simulink model "controlPosicion_2018a"  (R2018a)
settings: Solver=VariableStepAuto  StartTime=0.0  StopTime=18  RelTol=1e-3
values from neighbouring files (symbols this model uses):
  kp = 3    [Calculo_Tau_RR.m]
  kv = 2*sqrt(kp)    [Calculo_Tau_RR.m]
libraries: roblocks x5, simulink x1
settings Model: Creator=Marcelo  LastModifiedBy=rochi
settings DataIOCC: ReturnWorkspaceOutputs=on
settings SFSimCC: SimUseLocalCustomCode=on
settings RTWCC: RTWUseLocalCustomCode=on

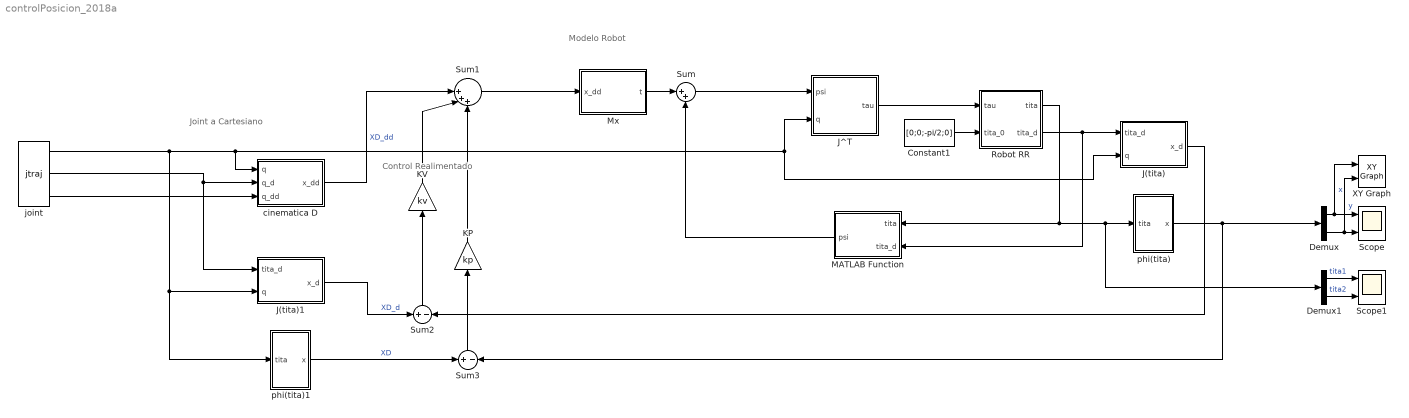
== system controlPosicion_2018a ==
  note: Control Realimentado
  note: Joint a Cartesiano
  note: Modelo Robot
  Constant1 : Constant  Value=[0;0;-pi/2;0]
  Demux : Demux  Outputs=2
  Demux1 : Demux  Outputs=2
  J(tita) : MATLAB Function  TreatAsAtomicUnit=on
  J(tita)1 : MATLAB Function  TreatAsAtomicUnit=on
  J^T : MATLAB Function  TreatAsAtomicUnit=on
  KP : Gain  Gain=kp
  KV : Gain  Gain=kv
  MATLAB Function : MATLAB Function  TreatAsAtomicUnit=on
  Mx : MATLAB Function  TreatAsAtomicUnit=on
  Robot RR : Subsystem
  Scope : Scope  NumInputPorts=2
  Scope1 : Scope  NumInputPorts=2
  Sum : Sum  Inputs=|++
  Sum1 : Sum  Inputs=||+++
  Sum2 : Sum  Inputs=+|-
  Sum3 : Sum  Inputs=+|-
  XY Graph : simulink/Sinks/XY Graph  xmin=-2  xmax=2  ymin=-2  ymax=2  st=-1
  cinematica D : MATLAB Function  TreatAsAtomicUnit=on
  joint : roblocks/Toolbox/jtraj  q0=[0 -pi/2]  qf=[pi/2 -pi/2]  tmax=10  ts=0.02
  phi(tita) : Subsystem
  phi(tita)1 : Subsystem
  wires:
  Robot RR/2(tita_d) -> J(tita)/1(tita_d), MATLAB Function/2(tita_d)
  MATLAB Function/1(psi) -> Sum/2
  KP/1 -> Sum1/3
  KV/1 -> Sum1/2
  Sum3/1 -> KP/1
  Sum2/1 -> KV/1
  phi(tita)/1(x) -> Sum3/2, Demux/1
  Demux/1 -> XY Graph/1, Scope/1  "x"
  Demux/2 -> XY Graph/2, Scope/2  "y"
  Constant1/1 -> Robot RR/2(tita_0)
  Mx/1(t) -> Sum/1
  Sum1/1 -> Mx/1(x_dd)
  Demux1/2 -> Scope1/2  "tita2"
  Demux1/1 -> Scope1/1  "tita1"
  J^T/1(tau) -> Robot RR/1(tau)
  Sum/1 -> J^T/1(psi)
  J(tita)/1(x_d) -> Sum2/2
  Robot RR/1(tita) -> Demux1/1, phi(tita)/1(tita), MATLAB Function/1(tita)
  joint/1 -> cinematica D/1(q), J(tita)/2(q), J^T/2(q), phi(tita)1/1(tita), J(tita)1/2(q)
  phi(tita)1/1(x) -> Sum3/1  "XD"
  J(tita)1/1(x_d) -> Sum2/1  "XD_d"
  joint/2 -> cinematica D/2(q_d), J(tita)1/1(tita_d)
  cinematica D/1(x_dd) -> Sum1/1  "XD_dd"
  joint/3 -> cinematica D/3(q_dd)

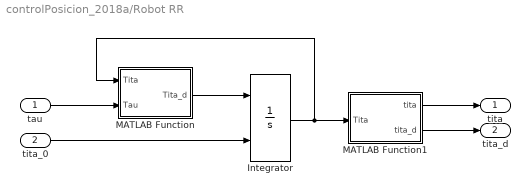
== system controlPosicion_2018a/Robot RR ==
  tau : Inport
  tita_0 : Inport  Port=2
  Integrator : Integrator  InitialConditionSource=external
  MATLAB Function : MATLAB Function  TreatAsAtomicUnit=on
  MATLAB Function1 : MATLAB Function  TreatAsAtomicUnit=on
  tita : Outport
  tita_d : Outport  Port=2
  wires:
  tau/1 -> MATLAB Function/2(Tau)
  MATLAB Function/1(Tita_d) -> Integrator/1
  tita_0/1 -> Integrator/2
  Integrator/1 -> MATLAB Function1/1(Tita), MATLAB Function/1(Tita)
  MATLAB Function1/1(tita) -> tita/1
  MATLAB Function1/2(tita_d) -> tita_d/1

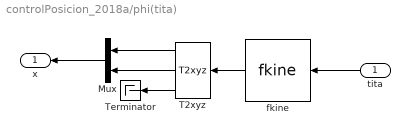
== system controlPosicion_2018a/phi(tita) ==
  tita : Inport
  Mux : Mux  Inputs=2
  T2xyz : roblocks/Toolbox/T2xyz
  Terminator : Terminator
  fkine : roblocks/Arm/fkine  robot=Robot
  x : Outport
  wires:
  T2xyz/2 -> Mux/2
  Mux/1 -> x/1
  fkine/1 -> T2xyz/1
  tita/1 -> fkine/1
  T2xyz/1 -> Mux/1
  T2xyz/3 -> Terminator/1

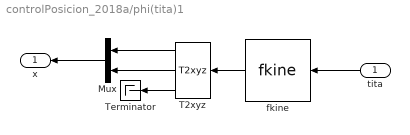
== system controlPosicion_2018a/phi(tita)1 ==
  tita : Inport
  Mux : Mux  Inputs=2
  T2xyz : roblocks/Toolbox/T2xyz
  Terminator : Terminator
  fkine : roblocks/Arm/fkine  robot=Robot
  x : Outport
  wires:
  T2xyz/2 -> Mux/2
  Mux/1 -> x/1
  fkine/1 -> T2xyz/1
  tita/1 -> fkine/1
  T2xyz/1 -> Mux/1
  T2xyz/3 -> Terminator/1

== matlab function controlPosicion_2018a/MATLAB Function ==
  data: tita input; psi output; tita_d input
function psi = f(tita,tita_d)

psi1 = tita_d(1);
psi2 = tita_d(2);

psi = [psi1;psi2];

== matlab function controlPosicion_2018a/J^T ==
  data: psi input; tau output; q input
function tau = fcn(psi,q)

th2 = q(2);
J = [sin(th2) 0; cos(th2)+1 1];

tau = (J')*psi;

== matlab function controlPosicion_2018a/Robot RR/MATLAB Function ==
  data: Tita input; Tita_d output; Tau input
function Tita_d = fcn(Tita,Tau)

titad1 = Tita(2);
titadd1 = Tau(1)-Tita(2);
titad2 = Tau(2);
titadd2 = 0;

Tita_d = [titad1;titadd1;titad2;titadd2];

== matlab function controlPosicion_2018a/Robot RR/MATLAB Function1 ==
  data: Tita input; tita output; tita_d output
function [tita,tita_d] = fcn(Tita)

tita = [Tita(1);Tita(3)];
tita_d = [Tita(2);Tita(4)];

== matlab function controlPosicion_2018a/J(tita)1 ==
  data: tita_d input; x_d output; q input
function x_d = fcn(tita_d,q)

th2 = q(2);
J = [sin(th2) 0; cos(th2)+1 1];

x_d = J*tita_d;

== matlab function controlPosicion_2018a/J(tita) ==
  data: tita_d input; x_d output; q input
function x_d = fcn(tita_d,q)

th2 = q(2);
J = [sin(th2) 0; cos(th2)+1 1];

x_d = J*tita_d;

== matlab function controlPosicion_2018a/cinematica D ==
  data: q input; x_dd output; q_d input; q_dd input
function x_dd = fcn(q,q_d,q_dd)

th2 = q(2);
th2_d = q_d(2);
J = [sin(th2) 0; cos(th2)+1 1];
J_d = [cos(th2)*th2_d 0;-sin(th2)*th2_d 0];

x_dd = J_d*q_d + J*q_dd;

== matlab function controlPosicion_2018a/Mx ==
  data: x_dd input; t output
function t = fcn(x_dd)

t = [x_dd(1);0];
